simulink model "BicycleModelAccelV2"  (R2021b)
settings: Solver=VariableStepAuto  StartTime=0.0  StopTime=10.0  RelTol=1e-3
settings Model: Creator=Pratham  LastModifiedBy=jpchi

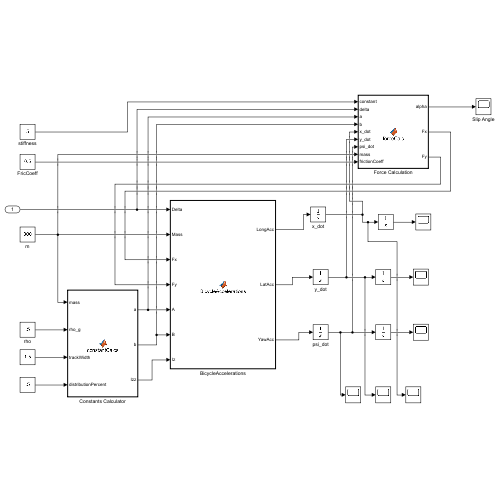
[thumbnail: Simulink's stored preview of the top-level diagram]
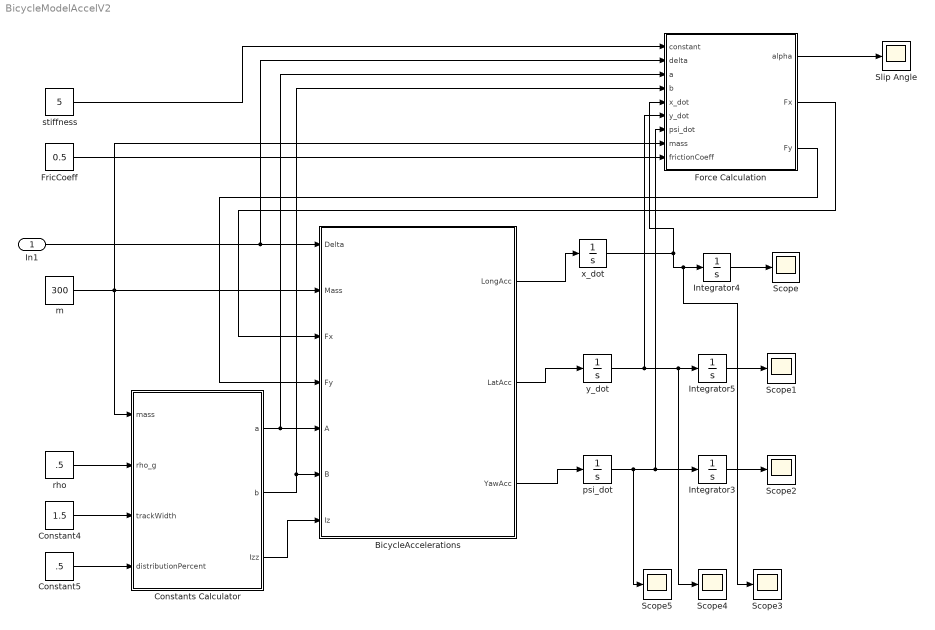
== system BicycleModelAccelV2 ==
  In1 : Inport
  BicycleAccelerations : MATLAB Function  TreatAsAtomicUnit=on
  Constant4 : Constant  Value=1.5
  Constant5 : Constant  Value=.5
  Constants Calculator : MATLAB Function  TreatAsAtomicUnit=on
  Force Calculation : MATLAB Function  TreatAsAtomicUnit=on
  FricCoeff : Constant  Value=0.5
  Integrator3 : Integrator
  Integrator4 : Integrator
  Integrator5 : Integrator
  Scope{,1..5} (6 alike) : Scope
  Slip Angle : Scope
  m : Constant  Value=300
  psi_dot : Integrator
  rho : Constant  Value=.5
  stiffness : Constant  Value=5
  x_dot : Integrator  InitialCondition=10
  y_dot : Integrator
  wires:
  BicycleAccelerations/2(LatAcc) -> y_dot/1
  BicycleAccelerations/3(YawAcc) -> psi_dot/1
  In1/1 -> Force Calculation/2(delta), BicycleAccelerations/1(Delta)
  m/1 -> Force Calculation/8(mass), BicycleAccelerations/2(Mass), Constants Calculator/1(mass)
  rho/1 -> Constants Calculator/2(rho_g)
  Constants Calculator/1(a) -> Force Calculation/3(a), BicycleAccelerations/5(A)
  Constants Calculator/2(b) -> Force Calculation/4(b), BicycleAccelerations/6(B)
  Constants Calculator/3(Izz) -> BicycleAccelerations/7(Iz)
  Constant4/1 -> Constants Calculator/3(trackWidth)
  Constant5/1 -> Constants Calculator/4(distributionPercent)
  Integrator3/1 -> Scope2/1
  Integrator5/1 -> Scope1/1
  y_dot/1 -> Force Calculation/6(y_dot), Scope4/1, Integrator5/1
  psi_dot/1 -> Scope5/1, Force Calculation/7(psi_dot), Integrator3/1
  Force Calculation/2(Fx) -> BicycleAccelerations/3(Fx)
  Force Calculation/3(Fy) -> BicycleAccelerations/4(Fy)
  Force Calculation/1(alpha) -> Slip Angle/1
  FricCoeff/1 -> Force Calculation/9(frictionCoeff)
  stiffness/1 -> Force Calculation/1(constant)
  Integrator4/1 -> Scope/1
  x_dot/1 -> Scope3/1, Integrator4/1, Force Calculation/5(x_dot)
  BicycleAccelerations/1(LongAcc) -> x_dot/1

== matlab function BicycleModelAccelV2/Constants Calculator ==
  data: a output; b output; mass input; Izz output; rho_g input; trackWidth input; distributionPercent input
function [a, b, Izz] = constantCalcs(mass, rho_g, trackWidth, distributionPercent)
Izz = mass*(rho_g)^2;
a = trackWidth*distributionPercent;
b = trackWidth - a;
end

== matlab function BicycleModelAccelV2/BicycleAccelerations ==
  data: LongAcc output; LatAcc output; Delta input; Mass input; YawAcc output; Fx input size=2; Fy input size=2; A input; B input; Iz input
function [LongAcc, LatAcc, YawAcc] = BicycleAccelerations (Delta, Mass, ...
    Fx, Fy, A, B, Iz)

%% BA - Bicycle Accelerations Calculations
% 
% Inputs:
%  Delta   - (n,1 numeric) Lateral Acceleration        {y_ddot} [m/s^2]
%  Mass    - (n,1 numeric) Mass                        {m}      [kg]
%  Fx      - (n,2 numeric) Force X-Direction           {F_x}    [kg*m/s^2]
%  Fy      - (n,2 numeric) Force Y-Direction           {F_y}    [kg*m/s^2]
%  A       - (n,1 numeric) Length C.O.M to Front Tire  {lf}     [m]
%  B       - (n,1 numeric) Length C.O.M to Back Tire   {lb}     [m]
%  Iz      - (n,1 numeric) Yaw Moment of Inertia       {I_z}    [kg*m^2]
%
% Outputs:
%  LatAcc  - (n,1 numeric) Lateral Acceleration        {y_ddot} [m/s^2]
%  LongAcc - (n,1 numeric) Longitudinal Acceleration   {x_ddot} [m/s^2]
%  YawAcc  - (n,1 numeric) Yaw Acceleration            {x_dot}  [m/s]
%  
% Notes:
% N/A
%
% Author(s): 
% Pratham Goradia (prgoradia@ucdavis.edu) [Aug 2021 - Sep 2021] 

% Last Updated: 21-Sep-2021

%% Test Cases
if nargin == 0
    %%% Test Inputs
    %Delta = 15; 
    
    %Mass = 300; 
    %A = 2;
    %B = 3;
    
    %Fx = [10, 10];
    %Fy = [10,10];
    %Iz = 5;
  
    
    %fprintf('Executing Bicycle Accelerations() Test Cases: \n');
    
    
    %[LongAcc, LatAcc, YawAcc] = BicycleAccelerations (Delta, Mass, Fx, Fy, A, B, Iz);
    
    
        
end
    
%% Computation

% Accelerations
LongAcc = (Fx(1)*cosd(Delta) - Fy(1)*sind(Delta) + Fx(2))/Mass;
LatAcc = (Fy(1)*cosd(Delta) + Fx(1)*sind(Delta) + Fy(2))/Mass;
YawAcc = (A*(Fy(1)*cosd(Delta) + Fx(1)*sind(Delta)) - B*Fy(2))/Iz;
end

== matlab function BicycleModelAccelV2/Force Calculation ==
  data: constant input; delta input; alpha output size=[1 2]; a input; b input; x_dot input; y_dot input; psi_dot input; Fx output size=[1 2]; Fy output size=[1 2]; mass input; frictionCoeff input
function [alpha, Fx, Fy]  = forceCalc(constant, delta, a, ... 
b, x_dot, y_dot, psi_dot, mass, frictionCoeff)
grav = 9.81;
alpha = zeros(1,2);
Fx = zeros(1,2);
Fy = zeros(1,2);
alpha(1) = delta - atand(y_dot + a.*psi_dot ./ x_dot);
alpha(2) = -atand(y_dot - b.*psi_dot ./ x_dot);
Fx(1) = constant.*alpha(1) + mass.*grav.*frictionCoeff;
Fy(1) = constant.*alpha(2) + mass.*grav.*frictionCoeff;
end
